simulink model "DA40_Flight_Model"  (R2023a)
settings: Solver=FixedStepAuto  StartTime=DCAM.startTime  StopTime=DCAM.endTime  FixedStep=DCAM.timeStep  RelTol=1e-3
undefined symbols (not defined in the file or in its folder): DCAM, Earth, WGS84
libraries: simulink x27, slpidlib x15, simulink_extras x6, sharedtransform x4, aerolibtransform2 x4, aerolibatmos2 x3, uavalgslib x2, aerolibwind2 x1
(part 2 of 6)

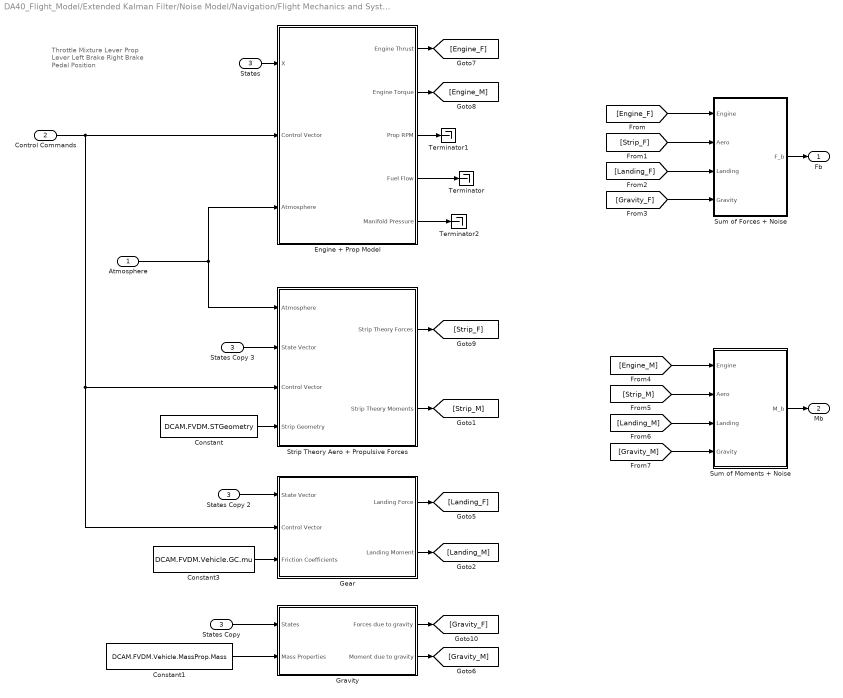
== system DA40_Flight_Model/Extended Kalman Filter/Noise Model/Navigation/Flight Mechanics and Systems Models ==
  note: Throttle
      | Mixture Lever
      | Prop Lever
      | Left Brake
      | Right Brake
      | Pedal Position
  Atmosphere : Inport
  Control Commands : Inport  Port=2
  States : Inport  Port=3
  Constant : Constant  Value=DCAM.FVDM.STGeometry
  Constant1 : Constant  Value=DCAM.FVDM.Vehicle.MassProp.Mass
  Constant3 : Constant  Value=DCAM.FVDM.Vehicle.GC.mu
  Engine + Prop Model : Subsystem
  Gear : Subsystem
  Gravity : Subsystem
  States Copy : InportShadow  Port=3
  States Copy 2 : InportShadow  Port=3
  States Copy 3 : InportShadow  Port=3
  Strip Theory Aero + Propulsive Forces : Subsystem
  Sum of Forces + Noise : Subsystem
  Sum of Moments + Noise : Subsystem
  Terminator : Terminator
  Terminator1 : Terminator
  Terminator2 : Terminator
  Fb : Outport
  Mb : Outport  Port=2
  wires:
  States/1 -> Engine + Prop Model/1(X)
  Constant1/1 -> Gravity/2(Mass Properties)
  Constant/1 -> Strip Theory Aero + Propulsive Forces/4(Strip Geometry)
  Engine + Prop Model/5(Manifold Pressure) -> Terminator2/1
  Engine + Prop Model/3(Prop RPM) -> Terminator1/1
  Constant3/1 -> Gear/3(Friction Coefficients)
  States Copy/1 -> Gravity/1(States)
  States Copy 2/1 -> Gear/1(State Vector)
  States Copy 3/1 -> Strip Theory Aero + Propulsive Forces/2(State Vector)
  Control Commands/1 -> Strip Theory Aero + Propulsive Forces/3(Control Vector), Gear/2(Control Vector), Engine + Prop Model/2(Control Vector)
  Engine + Prop Model/2(Engine Torque) -> [Engine_M]
  Strip Theory Aero + Propulsive Forces/2(Strip Theory Moments) -> [Strip_M]
  Gear/2(Landing Moment) -> [Landing_M]
  Gravity/2(Moment due to gravity) -> [Gravity_M]
  Gravity/1(Forces due to gravity) -> [Gravity_F]
  Gear/1(Landing Force) -> [Landing_F]
  Strip Theory Aero + Propulsive Forces/1(Strip Theory Forces) -> [Strip_F]
  Engine + Prop Model/1(Engine Thrust) -> [Engine_F]
  Sum of Forces + Noise/1(F_b) -> Fb/1
  [Engine_M] -> Sum of Moments + Noise/1(Engine)
  [Strip_M] -> Sum of Moments + Noise/2(Aero)
  [Landing_M] -> Sum of Moments + Noise/3(Landing)
  [Gravity_M] -> Sum of Moments + Noise/4(Gravity)
  Atmosphere/1 -> Strip Theory Aero + Propulsive Forces/1(Atmosphere), Engine + Prop Model/3(Atmosphere)
  Engine + Prop Model/4(Fuel Flow) -> Terminator/1
  [Gravity_F] -> Sum of Forces + Noise/4(Gravity)
  [Landing_F] -> Sum of Forces + Noise/3(Landing)
  [Strip_F] -> Sum of Forces + Noise/2(Aero)
  [Engine_F] -> Sum of Forces + Noise/1(Engine)
  Sum of Moments + Noise/1(M_b) -> Mb/1

== system DA40_Flight_Model/Correlator Simulation/Subsystem1/Generating GPS and Satellite Measurements/Truth Model/Control ==
  Commands : Inport
  States : Inport  Port=2
  Atmos : Inport  Port=3
  Bus Creator : BusCreator  Inputs=12
  Bus Selector : BusSelector  OutputSignals=Commanded Pitch,Commanded Bank,Commanded Velocity,Commanded Propeller Efficiency,Commanded Fuel Mixture,Commanded Flap Angle,Commanded Left Brake,Commanded Right Brake,Commanded Aileron Trim,Commanded Elevator Trim,Commanded Rudder Trim
  Send To Workspace : Subsystem
      settings: PortSchema="{\"entries\":[{\"content\":{\"sides\":[{\"content\":{\"connectorIds\":[\"In1\"]},\"type\":\"ConnectorPlacement.EquallySpacedRectSide\",\"uuid\":\"f8d70518-feba-4467-9144-e72499141e10\"},{\"content\":{\"connectorIds\":[\"Out1\"],\"side\":\"RIGHT\"},\"type\":\"ConnectorPlacement.EquallySpacedRectSide\",\"uuid\":\"0d837ca8-6650-40ee-933a-3521e14176de\"},{\"content\":{\"side\":\"TOP\"},\"type\":\"ConnectorPlacement.EquallySpacedRectSide\",\"uuid\":\"54f7b60b-7724-46f0-8f38-219401d515c7\"},{\"content\":{\"connectorIds\":[\"Out2\"],\"side\":\"BOTTOM\"},\"type\":\"ConnectorPlacement.EquallySpacedRectSide\",\"uuid\":\"f1e71b5c-4796-4085-9245-75f71ccb39d6\"}]},\"type\":\"ConnectorPlacement.EquallySpacedConnector\",\"uuid\":\"946e06f8-2adb-45c5-9153-0b4b2f8d0bb6\"}],\"packageUris\":[\"http://schema.mathworks.com/mf0/Connector/R2020b\"],\"version\":\"1.0\"}"
  Subsystem : Subsystem
      settings: PortSchema="{\"entries\":[{\"content\":{\"sides\":[{\"content\":{\"connectorIds\":[\"In1\"]},\"type\":\"ConnectorPlacement.EquallySpacedRectSide\",\"uuid\":\"5ea7349d-baf6-49c5-809d-4b912ce56d76\"},{\"content\":{\"connectorIds\":[\"Out1\",\"Out2\"],\"side\":\"RIGHT\"},\"type\":\"ConnectorPlacement.EquallySpacedRectSide\",\"uuid\":\"ab3ceec7-e245-42b0-9eb8-e3a68951e219\"},{\"content\":{\"connectorIds\":[\"In2\"],\"side\":\"TOP\"},\"type\":\"ConnectorPlacement.EquallySpacedRectSide\",\"uuid\":\"18178c43-0035-4aec-a3ba-011af3830f5c\"},{\"content\":{\"connectorIds\":[\"Out3\"],\"side\":\"BOTTOM\"},\"type\":\"ConnectorPlacement.EquallySpacedRectSide\",\"uuid\":\"88476787-2df8-4308-98f2-16231590cef9\"}]},\"type\":\"ConnectorPlacement.EquallySpacedConnector\",\"uuid\":\"0f7476f8-a4e6-4d2f-9698-249fd1b1cc90\"}],\"packageUris\":[\"http://schema.mathworks.com/mf0/Connector/R2020b\"],\"version\":\"1.0\"}"
  Subsystem1 : Subsystem
      settings: PortSchema="{\"entries\":[{\"content\":{\"sides\":[{\"content\":{\"connectorIds\":[\"In1\"]},\"type\":\"ConnectorPlacement.EquallySpacedRectSide\",\"uuid\":\"df1e81ab-d97f-43f0-8cd1-ba06c25288e8\"},{\"content\":{\"connectorIds\":[\"Out1\"],\"side\":\"RIGHT\"},\"type\":\"ConnectorPlacement.EquallySpacedRectSide\",\"uuid\":\"fe7f65be-8a13-42ab-8ffa-afe418a633fa\"},{\"content\":{\"connectorIds\":[\"In2\"],\"side\":\"TOP\"},\"type\":\"ConnectorPlacement.EquallySpacedRectSide\",\"uuid\":\"4762097a-1dfd-4646-aeb3-678774417eb9\"},{\"content\":{\"connectorIds\":[\"Out2\"],\"side\":\"BOTTOM\"},\"type\":\"ConnectorPlacement.EquallySpacedRectSide\",\"uuid\":\"338e28fc-4594-4f48-8379-f1c16de78061\"}]},\"type\":\"ConnectorPlacement.EquallySpacedConnector\",\"uuid\":\"e1e6a329-5243-44ef-b6a4-a2802fff17f2\"}],\"packageUris\":[\"http://schema.mathworks.com/mf0/Connector/R2020b\"],\"version\":\"1.0\"}"
  Subsystem10 : Subsystem
      settings: PortSchema="{\"entries\":[{\"content\":{\"sides\":[{\"content\":{\"connectorIds\":[\"In1\"]},\"type\":\"ConnectorPlacement.EquallySpacedRectSide\",\"uuid\":\"df1e81ab-d97f-43f0-8cd1-ba06c25288e8\"},{\"content\":{\"connectorIds\":[\"Out1\"],\"side\":\"RIGHT\"},\"type\":\"ConnectorPlacement.EquallySpacedRectSide\",\"uuid\":\"fe7f65be-8a13-42ab-8ffa-afe418a633fa\"},{\"content\":{\"connectorIds\":[\"In2\"],\"side\":\"TOP\"},\"type\":\"ConnectorPlacement.EquallySpacedRectSide\",\"uuid\":\"4762097a-1dfd-4646-aeb3-678774417eb9\"},{\"content\":{\"connectorIds\":[\"Out2\"],\"side\":\"BOTTOM\"},\"type\":\"ConnectorPlacement.EquallySpacedRectSide\",\"uuid\":\"ca232b1a-28ac-4e7a-b8a6-76103b2c6113\"}]},\"type\":\"ConnectorPlacement.EquallySpacedConnector\",\"uuid\":\"e1e6a329-5243-44ef-b6a4-a2802fff17f2\"}],\"packageUris\":[\"http://schema.mathworks.com/mf0/Connector/R2020b\"],\"version\":\"1.0\"}"
  Subsystem11 : Subsystem
      settings: PortSchema="{\"entries\":[{\"content\":{\"sides\":[{\"content\":{\"connectorIds\":[\"In1\"]},\"type\":\"ConnectorPlacement.EquallySpacedRectSide\",\"uuid\":\"df1e81ab-d97f-43f0-8cd1-ba06c25288e8\"},{\"content\":{\"connectorIds\":[\"Out1\"],\"side\":\"RIGHT\"},\"type\":\"ConnectorPlacement.EquallySpacedRectSide\",\"uuid\":\"fe7f65be-8a13-42ab-8ffa-afe418a633fa\"},{\"content\":{\"connectorIds\":[\"In2\"],\"side\":\"TOP\"},\"type\":\"ConnectorPlacement.EquallySpacedRectSide\",\"uuid\":\"4762097a-1dfd-4646-aeb3-678774417eb9\"}]},\"type\":\"ConnectorPlacement.EquallySpacedConnector\",\"uuid\":\"e1e6a329-5243-44ef-b6a4-a2802fff17f2\"}],\"packageUris\":[\"http://schema.mathworks.com/mf0/Connector/R2020b\"],\"version\":\"1.0\"}"
  Subsystem3 : Subsystem
      settings: PortSchema="{\"entries\":[{\"content\":{\"sides\":[{\"content\":{\"connectorIds\":[\"In1\"]},\"type\":\"ConnectorPlacement.EquallySpacedRectSide\",\"uuid\":\"df1e81ab-d97f-43f0-8cd1-ba06c25288e8\"},{\"content\":{\"connectorIds\":[\"Out1\"],\"side\":\"RIGHT\"},\"type\":\"ConnectorPlacement.EquallySpacedRectSide\",\"uuid\":\"fe7f65be-8a13-42ab-8ffa-afe418a633fa\"},{\"content\":{\"connectorIds\":[\"In2\"],\"side\":\"TOP\"},\"type\":\"ConnectorPlacement.EquallySpacedRectSide\",\"uuid\":\"4762097a-1dfd-4646-aeb3-678774417eb9\"},{\"content\":{\"connectorIds\":[\"Out2\"],\"side\":\"BOTTOM\"},\"type\":\"ConnectorPlacement.EquallySpacedRectSide\",\"uuid\":\"eb7acd08-7b98-4b28-a61a-3ca4385205ec\"}]},\"type\":\"ConnectorPlacement.EquallySpacedConnector\",\"uuid\":\"e1e6a329-5243-44ef-b6a4-a2802fff17f2\"}],\"packageUris\":[\"http://schema.mathworks.com/mf0/Connector/R2020b\"],\"version\":\"1.0\"}"
  Subsystem4 : Subsystem
      settings: PortSchema="{\"entries\":[{\"content\":{\"sides\":[{\"content\":{\"connectorIds\":[\"In1\"]},\"type\":\"ConnectorPlacement.EquallySpacedRectSide\",\"uuid\":\"df1e81ab-d97f-43f0-8cd1-ba06c25288e8\"},{\"content\":{\"connectorIds\":[\"Out1\"],\"side\":\"RIGHT\"},\"type\":\"ConnectorPlacement.EquallySpacedRectSide\",\"uuid\":\"fe7f65be-8a13-42ab-8ffa-afe418a633fa\"},{\"content\":{\"connectorIds\":[\"In2\"],\"side\":\"TOP\"},\"type\":\"ConnectorPlacement.EquallySpacedRectSide\",\"uuid\":\"4762097a-1dfd-4646-aeb3-678774417eb9\"},{\"content\":{\"connectorIds\":[\"Out2\"],\"side\":\"BOTTOM\"},\"type\":\"ConnectorPlacement.EquallySpacedRectSide\",\"uuid\":\"aca1bd27-9370-4c71-9435-0c269f9a438b\"}]},\"type\":\"ConnectorPlacement.EquallySpacedConnector\",\"uuid\":\"e1e6a329-5243-44ef-b6a4-a2802fff17f2\"}],\"packageUris\":[\"http://schema.mathworks.com/mf0/Connector/R2020b\"],\"version\":\"1.0\"}"
  Subsystem5 : Subsystem
      settings: PortSchema="{\"entries\":[{\"content\":{\"sides\":[{\"content\":{\"connectorIds\":[\"In1\"]},\"type\":\"ConnectorPlacement.EquallySpacedRectSide\",\"uuid\":\"df1e81ab-d97f-43f0-8cd1-ba06c25288e8\"},{\"content\":{\"connectorIds\":[\"Out1\"],\"side\":\"RIGHT\"},\"type\":\"ConnectorPlacement.EquallySpacedRectSide\",\"uuid\":\"fe7f65be-8a13-42ab-8ffa-afe418a633fa\"},{\"content\":{\"connectorIds\":[\"In2\"],\"side\":\"TOP\"},\"type\":\"ConnectorPlacement.EquallySpacedRectSide\",\"uuid\":\"4762097a-1dfd-4646-aeb3-678774417eb9\"},{\"content\":{\"connectorIds\":[\"Out2\"],\"side\":\"BOTTOM\"},\"type\":\"ConnectorPlacement.EquallySpacedRectSide\",\"uuid\":\"e3132084-5e8e-4693-9249-2c258902bcf1\"}]},\"type\":\"ConnectorPlacement.EquallySpacedConnector\",\"uuid\":\"e1e6a329-5243-44ef-b6a4-a2802fff17f2\"}],\"packageUris\":[\"http://schema.mathworks.com/mf0/Connector/R2020b\"],\"version\":\"1.0\"}"
  Subsystem6 : Subsystem
      settings: PortSchema="{\"entries\":[{\"content\":{\"sides\":[{\"content\":{\"connectorIds\":[\"In1\"]},\"type\":\"ConnectorPlacement.EquallySpacedRectSide\",\"uuid\":\"df1e81ab-d97f-43f0-8cd1-ba06c25288e8\"},{\"content\":{\"connectorIds\":[\"Out1\"],\"side\":\"RIGHT\"},\"type\":\"ConnectorPlacement.EquallySpacedRectSide\",\"uuid\":\"fe7f65be-8a13-42ab-8ffa-afe418a633fa\"},{\"content\":{\"connectorIds\":[\"In2\"],\"side\":\"TOP\"},\"type\":\"ConnectorPlacement.EquallySpacedRectSide\",\"uuid\":\"4762097a-1dfd-4646-aeb3-678774417eb9\"},{\"content\":{\"connectorIds\":[\"Out2\"],\"side\":\"BOTTOM\"},\"type\":\"ConnectorPlacement.EquallySpacedRectSide\",\"uuid\":\"44b8b4cf-3de4-40e9-9bc3-b7b2ed15b9c4\"}]},\"type\":\"ConnectorPlacement.EquallySpacedConnector\",\"uuid\":\"e1e6a329-5243-44ef-b6a4-a2802fff17f2\"}],\"packageUris\":[\"http://schema.mathworks.com/mf0/Connector/R2020b\"],\"version\":\"1.0\"}"
  Subsystem7 : Subsystem
      settings: PortSchema="{\"entries\":[{\"content\":{\"sides\":[{\"content\":{\"connectorIds\":[\"In1\"]},\"type\":\"ConnectorPlacement.EquallySpacedRectSide\",\"uuid\":\"df1e81ab-d97f-43f0-8cd1-ba06c25288e8\"},{\"content\":{\"connectorIds\":[\"Out1\"],\"side\":\"RIGHT\"},\"type\":\"ConnectorPlacement.EquallySpacedRectSide\",\"uuid\":\"fe7f65be-8a13-42ab-8ffa-afe418a633fa\"},{\"content\":{\"connectorIds\":[\"In2\"],\"side\":\"TOP\"},\"type\":\"ConnectorPlacement.EquallySpacedRectSide\",\"uuid\":\"4762097a-1dfd-4646-aeb3-678774417eb9\"},{\"content\":{\"connectorIds\":[\"Out2\"],\"side\":\"BOTTOM\"},\"type\":\"ConnectorPlacement.EquallySpacedRectSide\",\"uuid\":\"4aea28e3-05ae-492c-9523-17787d8052fd\"}]},\"type\":\"ConnectorPlacement.EquallySpacedConnector\",\"uuid\":\"e1e6a329-5243-44ef-b6a4-a2802fff17f2\"}],\"packageUris\":[\"http://schema.mathworks.com/mf0/Connector/R2020b\"],\"version\":\"1.0\"}"
  Subsystem8 : Subsystem
      settings: PortSchema="{\"entries\":[{\"content\":{\"sides\":[{\"content\":{\"connectorIds\":[\"In1\"]},\"type\":\"ConnectorPlacement.EquallySpacedRectSide\",\"uuid\":\"df1e81ab-d97f-43f0-8cd1-ba06c25288e8\"},{\"content\":{\"connectorIds\":[\"Out1\"],\"side\":\"RIGHT\"},\"type\":\"ConnectorPlacement.EquallySpacedRectSide\",\"uuid\":\"fe7f65be-8a13-42ab-8ffa-afe418a633fa\"},{\"content\":{\"connectorIds\":[\"In2\"],\"side\":\"TOP\"},\"type\":\"ConnectorPlacement.EquallySpacedRectSide\",\"uuid\":\"4762097a-1dfd-4646-aeb3-678774417eb9\"},{\"content\":{\"connectorIds\":[\"Out2\"],\"side\":\"BOTTOM\"},\"type\":\"ConnectorPlacement.EquallySpacedRectSide\",\"uuid\":\"60b425fe-182c-41c2-bc4c-aa97cb3d7ccf\"}]},\"type\":\"ConnectorPlacement.EquallySpacedConnector\",\"uuid\":\"e1e6a329-5243-44ef-b6a4-a2802fff17f2\"}],\"packageUris\":[\"http://schema.mathworks.com/mf0/Connector/R2020b\"],\"version\":\"1.0\"}"
  Subsystem9 : Subsystem
      settings: PortSchema="{\"entries\":[{\"content\":{\"sides\":[{\"content\":{\"connectorIds\":[\"In1\"]},\"type\":\"ConnectorPlacement.EquallySpacedRectSide\",\"uuid\":\"df1e81ab-d97f-43f0-8cd1-ba06c25288e8\"},{\"content\":{\"connectorIds\":[\"Out1\"],\"side\":\"RIGHT\"},\"type\":\"ConnectorPlacement.EquallySpacedRectSide\",\"uuid\":\"fe7f65be-8a13-42ab-8ffa-afe418a633fa\"},{\"content\":{\"connectorIds\":[\"In2\"],\"side\":\"TOP\"},\"type\":\"ConnectorPlacement.EquallySpacedRectSide\",\"uuid\":\"4762097a-1dfd-4646-aeb3-678774417eb9\"},{\"content\":{\"connectorIds\":[\"Out2\"],\"side\":\"BOTTOM\"},\"type\":\"ConnectorPlacement.EquallySpacedRectSide\",\"uuid\":\"88e2b07d-9cf7-412b-8368-04827ebf702b\"}]},\"type\":\"ConnectorPlacement.EquallySpacedConnector\",\"uuid\":\"e1e6a329-5243-44ef-b6a4-a2802fff17f2\"}],\"packageUris\":[\"http://schema.mathworks.com/mf0/Connector/R2020b\"],\"version\":\"1.0\"}"
  To Workspace : ToWorkspace  VariableName=controls  SampleTime=-1
      settings: Save2DSignal=2-D array (concatenate along first dimension)
  Controls : Outport
  Atmosphere : Outport  Port=2
  LLA : Outport  Port=3
  wires:
  Subsystem11/1(Out1) -> Bus Creator/12  "RUDDER TRIM"
  Subsystem9/1(Out1) -> Bus Creator/10  "AILERON TRIM"
  Subsystem1/1(Longitudinal Stick) -> Bus Creator/1  "Longitudinal Stick"
  Subsystem/1(Lateral Stick) -> Bus Creator/2  "Lateral Stick"
  Subsystem6/1(Out1) -> Bus Creator/7  "FLAP ANGLE"
  Subsystem5/1(Out1) -> Bus Creator/6  "Mixture Lever"
  Subsystem3/1(Out1) -> Bus Creator/4  "Throttle"
  Subsystem8/1(Out1) -> Bus Creator/9  "RightBrake"
  Subsystem/2(Pedal Posn) -> Bus Creator/3  "Pedal Posn"
  Subsystem4/1(Out1) -> Bus Creator/5  "Prop Lever"
  Subsystem7/1(Out1) -> Bus Creator/8  "LeftBrake"
  Subsystem10/1(Out1) -> Bus Creator/11  "ELEVATOR TRIM"
  Bus Creator/1 -> To Workspace/1, Controls/1
  Commands/1 -> Bus Selector/1
  Bus Selector/11 -> Subsystem11/1(Reference)  "<Commanded Rudder Trim>"
  Bus Selector/10 -> Subsystem10/1(Reference)  "<Commanded Elevator Trim>"
  Bus Selector/9 -> Subsystem9/1(Reference)  "<Commanded Aileron Trim>"
  Bus Selector/8 -> Subsystem8/1(Reference)  "<Commanded Right Brake>"
  Bus Selector/7 -> Subsystem7/1(Reference)  "<Commanded Left Brake>"
  Bus Selector/6 -> Subsystem6/1(Reference)  "<Commanded Flap Angle>"
  Bus Selector/5 -> Subsystem5/1(Reference)  "<Commanded Fuel Mixture>"
  Bus Selector/4 -> Subsystem4/1(Reference)  "<Commanded Propeller Efficiency>"
  Bus Selector/3 -> Subsystem3/1(Reference)  "<Commanded Velocity>"
  Bus Selector/1 -> Subsystem1/1(Reference)  "<Commanded Pitch>"
  Bus Selector/2 -> Subsystem/1(Reference)  "<Commanded Bank>"
  States/1 -> Send To Workspace/1(States)
  Send To Workspace/2(States Out) -> Subsystem1/2(States)
  Subsystem6/2(" ") -> Subsystem7/2(States)
  Subsystem9/2(" ") -> Subsystem10/2(States)
  Subsystem3/2(" ") -> Subsystem4/2(States)
  Subsystem/3(" ") -> Subsystem3/2(States)
  Subsystem1/2(" ") -> Subsystem/2(States)
  Subsystem7/2(" ") -> Subsystem8/2(States)
  Subsystem8/2(" ") -> Subsystem9/2(States)
  Subsystem5/2(" ") -> Subsystem6/2(States)
  Subsystem4/2(" ") -> Subsystem5/2(States)
  Subsystem10/2(" ") -> Subsystem11/2(States)
  Atmos/1 -> Atmosphere/1
  Send To Workspace/1(LLA) -> LLA/1

== system DA40_Flight_Model/Correlator Simulation/Subsystem1/Generating GPS and Satellite Measurements/Truth Model/Environment ==
  States : Inport
  LLA : Inport  Port=2
  Bus Creator : BusCreator  Inputs=5
  Clock : Clock
  Constant1 : Constant  Value=DCAM.FVDM.dayOfYear
  Gain1 : Gain  Gain=-1
  Horizontal Wind Model 14 : WindHWM14
  ISA Atmosphere Model : aerolibatmos2/ISA Atmosphere Model  custom=off  g=9.80665  gamma=1.4  R=287.0531  L=0.0065  h_trop=11000  h_strat=20000  rho0=1.225  P0=101325  T0=288.15  h0=0
  MATLAB Function : MATLAB Function  TreatAsAtomicUnit=on
  Selector1 : Selector  InputPortWidth=12  IndexOptions=Index vector (dialog)  Indices=[9]  OutputSizes=1
  States Out : Outport
  Atmos : Outport  Port=2
  wires:
  States/1 -> MATLAB Function/2(states), States Out/1, Selector1/1
  Selector1/1 -> Gain1/1
  ISA Atmosphere Model/2 -> Bus Creator/2  "Speed of Sound"
  ISA Atmosphere Model/3 -> Bus Creator/3  "Pressure"
  Bus Creator/1 -> Atmos/1
  ISA Atmosphere Model/1 -> Bus Creator/1  "Temperature"
  Gain1/1 -> ISA Atmosphere Model/1
  ISA Atmosphere Model/4 -> Bus Creator/4  "Density"
  LLA/1 -> Horizontal Wind Model 14/1
  Clock/1 -> Horizontal Wind Model 14/3
  Constant1/1 -> Horizontal Wind Model 14/2
  Horizontal Wind Model 14/1 -> MATLAB Function/1(windVectorNav)  "Wind Vector"
  MATLAB Function/1(windVectorBody) -> Bus Creator/5

== system DA40_Flight_Model/Correlator Simulation/Subsystem1/Generating GPS and Satellite Measurements/Truth Model/Guidance ==
  States : Inport
  Atmosphere : Inport  Port=2
  Bus Creator : BusCreator  Inputs=11
  Bus Selector : BusSelector  OutputSignals=x,y,z,psi
  Constant : Constant  Value=DCAM.FVDM.waypoints
  Constant1 : Constant  Value=DCAM.FVDM.lookaheadDist
  MATLAB Function : MATLAB Function  TreatAsAtomicUnit=on
  Mux : Mux
  Radians to Degrees : simulink_extras/Transformations/Radians to Degrees
  Subsystem : Subsystem
  Terminator : Terminator
  Terminator1 : Terminator
  Waypoint Follower : uavalgslib/Waypoint Follower  UAVType=fixed-wing  StartFrom=first  TransitionRadiusSource=internal  TransitionRadius=10  MinLookaheadDistance=0.1  YawInput=off  ShowCrossTrackErrorOutput=off  ShowStatusOutput=off  SimulateUsing=Code generation
  Commands : Outport
  States Out : Outport  Port=2
  Atmos : Outport  Port=3
  wires:
  Bus Creator/1 -> Commands/1
  Subsystem/1(Bank) -> Bus Creator/1  "Commanded Bank"
  Subsystem/2(Pitch) -> Bus Creator/2  "Commanded Pitch"
  Subsystem/3(Velocity) -> Bus Creator/3  "Commanded Velocity"
  Subsystem/4(Propeller Efficiency) -> Bus Creator/4  "Commanded Propeller Efficiency"
  Subsystem/5(Fuel Efficiency) -> Bus Creator/5  "Commanded Fuel Mixture"
  Subsystem/6(Flap Angle) -> Bus Creator/6  "Commanded Flap Angle"
  Subsystem/7(Left Brake) -> Bus Creator/7  "Commanded Left Brake"
  Subsystem/8(Right Brake) -> Bus Creator/8  "Commanded Right Brake"
  Subsystem/9(Aileron trim) -> Bus Creator/9  "Commanded Aileron Trim"
  Subsystem/10(Elevator Trim) -> Bus Creator/10  "Commanded Elevator Trim"
  Subsystem/11(Rudder Trim) -> Bus Creator/11  "Commanded Rudder Trim"
  States/1 -> Bus Selector/1, States Out/1
  Waypoint Follower/3 -> Terminator/1
  Waypoint Follower/4 -> Terminator1/1
  Constant/1 -> Waypoint Follower/2
  Constant1/1 -> Waypoint Follower/3
  Mux/1 -> Waypoint Follower/1
  Bus Selector/1 -> Mux/1  "<x>"
  Bus Selector/2 -> Mux/2  "<y>"
  Bus Selector/3 -> Mux/3  "<z>"
  Waypoint Follower/2 -> MATLAB Function/1("heading ")
  Atmosphere/1 -> Atmos/1
  Waypoint Follower/1 -> Subsystem/1(Target)
  MATLAB Function/1(heading) -> Subsystem/2(Desired Heading)
  Radians to Degrees/1 -> Mux/4, Subsystem/3(Heading)
  Bus Selector/4 -> Radians to Degrees/1  "<psi>"

== system DA40_Flight_Model/Correlator Simulation/Subsystem1/Generating GPS and Satellite Measurements/Truth Model/Navigation1 ==
  Atmosphere : Inport
  Controls : Inport  Port=2
  Constant1 : Constant  Value=DCAM.FVDM.Vehicle.MassProp.Mass
  DA-40 Equations of Motion : Subsystem
  Flight Mechanics and Systems Models : Subsystem
  States : Outport
  wires:
  Flight Mechanics and Systems Models/1(Fb) -> DA-40 Equations of Motion/1(Fb [lb])
  Flight Mechanics and Systems Models/2(Mb) -> DA-40 Equations of Motion/2(Mb [lb-ft])
  Controls/1 -> Flight Mechanics and Systems Models/2(Control Commands)
  Atmosphere/1 -> Flight Mechanics and Systems Models/1(Atmosphere)
  Constant1/1 -> DA-40 Equations of Motion/3(Mass Properties)
  DA-40 Equations of Motion/1(States) -> States/1, Flight Mechanics and Systems Models/3(States)

== system DA40_Flight_Model/Correlator Simulation/Subsystem1/Generating GPS and Satellite Measurements1/Truth Model/Control ==
  Commands : Inport
  States : Inport  Port=2
  Atmos : Inport  Port=3
  Bus Creator : BusCreator  Inputs=12
  Bus Selector : BusSelector  OutputSignals=Commanded Pitch,Commanded Bank,Commanded Velocity,Commanded Propeller Efficiency,Commanded Fuel Mixture,Commanded Flap Angle,Commanded Left Brake,Commanded Right Brake,Commanded Aileron Trim,Commanded Elevator Trim,Commanded Rudder Trim
  Send To Workspace : Subsystem
      settings: PortSchema="{\"entries\":[{\"content\":{\"sides\":[{\"content\":{\"connectorIds\":[\"In1\"]},\"type\":\"ConnectorPlacement.EquallySpacedRectSide\",\"uuid\":\"f8d70518-feba-4467-9144-e72499141e10\"},{\"content\":{\"connectorIds\":[\"Out1\"],\"side\":\"RIGHT\"},\"type\":\"ConnectorPlacement.EquallySpacedRectSide\",\"uuid\":\"0d837ca8-6650-40ee-933a-3521e14176de\"},{\"content\":{\"side\":\"TOP\"},\"type\":\"ConnectorPlacement.EquallySpacedRectSide\",\"uuid\":\"54f7b60b-7724-46f0-8f38-219401d515c7\"},{\"content\":{\"connectorIds\":[\"Out2\"],\"side\":\"BOTTOM\"},\"type\":\"ConnectorPlacement.EquallySpacedRectSide\",\"uuid\":\"f1e71b5c-4796-4085-9245-75f71ccb39d6\"}]},\"type\":\"ConnectorPlacement.EquallySpacedConnector\",\"uuid\":\"946e06f8-2adb-45c5-9153-0b4b2f8d0bb6\"}],\"packageUris\":[\"http://schema.mathworks.com/mf0/Connector/R2020b\"],\"version\":\"1.0\"}"
  Subsystem : Subsystem
      settings: PortSchema="{\"entries\":[{\"content\":{\"sides\":[{\"content\":{\"connectorIds\":[\"In1\"]},\"type\":\"ConnectorPlacement.EquallySpacedRectSide\",\"uuid\":\"5ea7349d-baf6-49c5-809d-4b912ce56d76\"},{\"content\":{\"connectorIds\":[\"Out1\",\"Out2\"],\"side\":\"RIGHT\"},\"type\":\"ConnectorPlacement.EquallySpacedRectSide\",\"uuid\":\"ab3ceec7-e245-42b0-9eb8-e3a68951e219\"},{\"content\":{\"connectorIds\":[\"In2\"],\"side\":\"TOP\"},\"type\":\"ConnectorPlacement.EquallySpacedRectSide\",\"uuid\":\"18178c43-0035-4aec-a3ba-011af3830f5c\"},{\"content\":{\"connectorIds\":[\"Out3\"],\"side\":\"BOTTOM\"},\"type\":\"ConnectorPlacement.EquallySpacedRectSide\",\"uuid\":\"88476787-2df8-4308-98f2-16231590cef9\"}]},\"type\":\"ConnectorPlacement.EquallySpacedConnector\",\"uuid\":\"0f7476f8-a4e6-4d2f-9698-249fd1b1cc90\"}],\"packageUris\":[\"http://schema.mathworks.com/mf0/Connector/R2020b\"],\"version\":\"1.0\"}"
  Subsystem1 : Subsystem
      settings: PortSchema="{\"entries\":[{\"content\":{\"sides\":[{\"content\":{\"connectorIds\":[\"In1\"]},\"type\":\"ConnectorPlacement.EquallySpacedRectSide\",\"uuid\":\"df1e81ab-d97f-43f0-8cd1-ba06c25288e8\"},{\"content\":{\"connectorIds\":[\"Out1\"],\"side\":\"RIGHT\"},\"type\":\"ConnectorPlacement.EquallySpacedRectSide\",\"uuid\":\"fe7f65be-8a13-42ab-8ffa-afe418a633fa\"},{\"content\":{\"connectorIds\":[\"In2\"],\"side\":\"TOP\"},\"type\":\"ConnectorPlacement.EquallySpacedRectSide\",\"uuid\":\"4762097a-1dfd-4646-aeb3-678774417eb9\"},{\"content\":{\"connectorIds\":[\"Out2\"],\"side\":\"BOTTOM\"},\"type\":\"ConnectorPlacement.EquallySpacedRectSide\",\"uuid\":\"338e28fc-4594-4f48-8379-f1c16de78061\"}]},\"type\":\"ConnectorPlacement.EquallySpacedConnector\",\"uuid\":\"e1e6a329-5243-44ef-b6a4-a2802fff17f2\"}],\"packageUris\":[\"http://schema.mathworks.com/mf0/Connector/R2020b\"],\"version\":\"1.0\"}"
  Subsystem10 : Subsystem
      settings: PortSchema="{\"entries\":[{\"content\":{\"sides\":[{\"content\":{\"connectorIds\":[\"In1\"]},\"type\":\"ConnectorPlacement.EquallySpacedRectSide\",\"uuid\":\"df1e81ab-d97f-43f0-8cd1-ba06c25288e8\"},{\"content\":{\"connectorIds\":[\"Out1\"],\"side\":\"RIGHT\"},\"type\":\"ConnectorPlacement.EquallySpacedRectSide\",\"uuid\":\"fe7f65be-8a13-42ab-8ffa-afe418a633fa\"},{\"content\":{\"connectorIds\":[\"In2\"],\"side\":\"TOP\"},\"type\":\"ConnectorPlacement.EquallySpacedRectSide\",\"uuid\":\"4762097a-1dfd-4646-aeb3-678774417eb9\"},{\"content\":{\"connectorIds\":[\"Out2\"],\"side\":\"BOTTOM\"},\"type\":\"ConnectorPlacement.EquallySpacedRectSide\",\"uuid\":\"ca232b1a-28ac-4e7a-b8a6-76103b2c6113\"}]},\"type\":\"ConnectorPlacement.EquallySpacedConnector\",\"uuid\":\"e1e6a329-5243-44ef-b6a4-a2802fff17f2\"}],\"packageUris\":[\"http://schema.mathworks.com/mf0/Connector/R2020b\"],\"version\":\"1.0\"}"
  Subsystem11 : Subsystem
      settings: PortSchema="{\"entries\":[{\"content\":{\"sides\":[{\"content\":{\"connectorIds\":[\"In1\"]},\"type\":\"ConnectorPlacement.EquallySpacedRectSide\",\"uuid\":\"df1e81ab-d97f-43f0-8cd1-ba06c25288e8\"},{\"content\":{\"connectorIds\":[\"Out1\"],\"side\":\"RIGHT\"},\"type\":\"ConnectorPlacement.EquallySpacedRectSide\",\"uuid\":\"fe7f65be-8a13-42ab-8ffa-afe418a633fa\"},{\"content\":{\"connectorIds\":[\"In2\"],\"side\":\"TOP\"},\"type\":\"ConnectorPlacement.EquallySpacedRectSide\",\"uuid\":\"4762097a-1dfd-4646-aeb3-678774417eb9\"}]},\"type\":\"ConnectorPlacement.EquallySpacedConnector\",\"uuid\":\"e1e6a329-5243-44ef-b6a4-a2802fff17f2\"}],\"packageUris\":[\"http://schema.mathworks.com/mf0/Connector/R2020b\"],\"version\":\"1.0\"}"
  Subsystem3 : Subsystem
      settings: PortSchema="{\"entries\":[{\"content\":{\"sides\":[{\"content\":{\"connectorIds\":[\"In1\"]},\"type\":\"ConnectorPlacement.EquallySpacedRectSide\",\"uuid\":\"df1e81ab-d97f-43f0-8cd1-ba06c25288e8\"},{\"content\":{\"connectorIds\":[\"Out1\"],\"side\":\"RIGHT\"},\"type\":\"ConnectorPlacement.EquallySpacedRectSide\",\"uuid\":\"fe7f65be-8a13-42ab-8ffa-afe418a633fa\"},{\"content\":{\"connectorIds\":[\"In2\"],\"side\":\"TOP\"},\"type\":\"ConnectorPlacement.EquallySpacedRectSide\",\"uuid\":\"4762097a-1dfd-4646-aeb3-678774417eb9\"},{\"content\":{\"connectorIds\":[\"Out2\"],\"side\":\"BOTTOM\"},\"type\":\"ConnectorPlacement.EquallySpacedRectSide\",\"uuid\":\"eb7acd08-7b98-4b28-a61a-3ca4385205ec\"}]},\"type\":\"ConnectorPlacement.EquallySpacedConnector\",\"uuid\":\"e1e6a329-5243-44ef-b6a4-a2802fff17f2\"}],\"packageUris\":[\"http://schema.mathworks.com/mf0/Connector/R2020b\"],\"version\":\"1.0\"}"
  Subsystem4 : Subsystem
      settings: PortSchema="{\"entries\":[{\"content\":{\"sides\":[{\"content\":{\"connectorIds\":[\"In1\"]},\"type\":\"ConnectorPlacement.EquallySpacedRectSide\",\"uuid\":\"df1e81ab-d97f-43f0-8cd1-ba06c25288e8\"},{\"content\":{\"connectorIds\":[\"Out1\"],\"side\":\"RIGHT\"},\"type\":\"ConnectorPlacement.EquallySpacedRectSide\",\"uuid\":\"fe7f65be-8a13-42ab-8ffa-afe418a633fa\"},{\"content\":{\"connectorIds\":[\"In2\"],\"side\":\"TOP\"},\"type\":\"ConnectorPlacement.EquallySpacedRectSide\",\"uuid\":\"4762097a-1dfd-4646-aeb3-678774417eb9\"},{\"content\":{\"connectorIds\":[\"Out2\"],\"side\":\"BOTTOM\"},\"type\":\"ConnectorPlacement.EquallySpacedRectSide\",\"uuid\":\"aca1bd27-9370-4c71-9435-0c269f9a438b\"}]},\"type\":\"ConnectorPlacement.EquallySpacedConnector\",\"uuid\":\"e1e6a329-5243-44ef-b6a4-a2802fff17f2\"}],\"packageUris\":[\"http://schema.mathworks.com/mf0/Connector/R2020b\"],\"version\":\"1.0\"}"
  Subsystem5 : Subsystem
      settings: PortSchema="{\"entries\":[{\"content\":{\"sides\":[{\"content\":{\"connectorIds\":[\"In1\"]},\"type\":\"ConnectorPlacement.EquallySpacedRectSide\",\"uuid\":\"df1e81ab-d97f-43f0-8cd1-ba06c25288e8\"},{\"content\":{\"connectorIds\":[\"Out1\"],\"side\":\"RIGHT\"},\"type\":\"ConnectorPlacement.EquallySpacedRectSide\",\"uuid\":\"fe7f65be-8a13-42ab-8ffa-afe418a633fa\"},{\"content\":{\"connectorIds\":[\"In2\"],\"side\":\"TOP\"},\"type\":\"ConnectorPlacement.EquallySpacedRectSide\",\"uuid\":\"4762097a-1dfd-4646-aeb3-678774417eb9\"},{\"content\":{\"connectorIds\":[\"Out2\"],\"side\":\"BOTTOM\"},\"type\":\"ConnectorPlacement.EquallySpacedRectSide\",\"uuid\":\"e3132084-5e8e-4693-9249-2c258902bcf1\"}]},\"type\":\"ConnectorPlacement.EquallySpacedConnector\",\"uuid\":\"e1e6a329-5243-44ef-b6a4-a2802fff17f2\"}],\"packageUris\":[\"http://schema.mathworks.com/mf0/Connector/R2020b\"],\"version\":\"1.0\"}"
  Subsystem6 : Subsystem
      settings: PortSchema="{\"entries\":[{\"content\":{\"sides\":[{\"content\":{\"connectorIds\":[\"In1\"]},\"type\":\"ConnectorPlacement.EquallySpacedRectSide\",\"uuid\":\"df1e81ab-d97f-43f0-8cd1-ba06c25288e8\"},{\"content\":{\"connectorIds\":[\"Out1\"],\"side\":\"RIGHT\"},\"type\":\"ConnectorPlacement.EquallySpacedRectSide\",\"uuid\":\"fe7f65be-8a13-42ab-8ffa-afe418a633fa\"},{\"content\":{\"connectorIds\":[\"In2\"],\"side\":\"TOP\"},\"type\":\"ConnectorPlacement.EquallySpacedRectSide\",\"uuid\":\"4762097a-1dfd-4646-aeb3-678774417eb9\"},{\"content\":{\"connectorIds\":[\"Out2\"],\"side\":\"BOTTOM\"},\"type\":\"ConnectorPlacement.EquallySpacedRectSide\",\"uuid\":\"44b8b4cf-3de4-40e9-9bc3-b7b2ed15b9c4\"}]},\"type\":\"ConnectorPlacement.EquallySpacedConnector\",\"uuid\":\"e1e6a329-5243-44ef-b6a4-a2802fff17f2\"}],\"packageUris\":[\"http://schema.mathworks.com/mf0/Connector/R2020b\"],\"version\":\"1.0\"}"
  Subsystem7 : Subsystem
      settings: PortSchema="{\"entries\":[{\"content\":{\"sides\":[{\"content\":{\"connectorIds\":[\"In1\"]},\"type\":\"ConnectorPlacement.EquallySpacedRectSide\",\"uuid\":\"df1e81ab-d97f-43f0-8cd1-ba06c25288e8\"},{\"content\":{\"connectorIds\":[\"Out1\"],\"side\":\"RIGHT\"},\"type\":\"ConnectorPlacement.EquallySpacedRectSide\",\"uuid\":\"fe7f65be-8a13-42ab-8ffa-afe418a633fa\"},{\"content\":{\"connectorIds\":[\"In2\"],\"side\":\"TOP\"},\"type\":\"ConnectorPlacement.EquallySpacedRectSide\",\"uuid\":\"4762097a-1dfd-4646-aeb3-678774417eb9\"},{\"content\":{\"connectorIds\":[\"Out2\"],\"side\":\"BOTTOM\"},\"type\":\"ConnectorPlacement.EquallySpacedRectSide\",\"uuid\":\"4aea28e3-05ae-492c-9523-17787d8052fd\"}]},\"type\":\"ConnectorPlacement.EquallySpacedConnector\",\"uuid\":\"e1e6a329-5243-44ef-b6a4-a2802fff17f2\"}],\"packageUris\":[\"http://schema.mathworks.com/mf0/Connector/R2020b\"],\"version\":\"1.0\"}"
  Subsystem8 : Subsystem
      settings: PortSchema="{\"entries\":[{\"content\":{\"sides\":[{\"content\":{\"connectorIds\":[\"In1\"]},\"type\":\"ConnectorPlacement.EquallySpacedRectSide\",\"uuid\":\"df1e81ab-d97f-43f0-8cd1-ba06c25288e8\"},{\"content\":{\"connectorIds\":[\"Out1\"],\"side\":\"RIGHT\"},\"type\":\"ConnectorPlacement.EquallySpacedRectSide\",\"uuid\":\"fe7f65be-8a13-42ab-8ffa-afe418a633fa\"},{\"content\":{\"connectorIds\":[\"In2\"],\"side\":\"TOP\"},\"type\":\"ConnectorPlacement.EquallySpacedRectSide\",\"uuid\":\"4762097a-1dfd-4646-aeb3-678774417eb9\"},{\"content\":{\"connectorIds\":[\"Out2\"],\"side\":\"BOTTOM\"},\"type\":\"ConnectorPlacement.EquallySpacedRectSide\",\"uuid\":\"60b425fe-182c-41c2-bc4c-aa97cb3d7ccf\"}]},\"type\":\"ConnectorPlacement.EquallySpacedConnector\",\"uuid\":\"e1e6a329-5243-44ef-b6a4-a2802fff17f2\"}],\"packageUris\":[\"http://schema.mathworks.com/mf0/Connector/R2020b\"],\"version\":\"1.0\"}"
  Subsystem9 : Subsystem
      settings: PortSchema="{\"entries\":[{\"content\":{\"sides\":[{\"content\":{\"connectorIds\":[\"In1\"]},\"type\":\"ConnectorPlacement.EquallySpacedRectSide\",\"uuid\":\"df1e81ab-d97f-43f0-8cd1-ba06c25288e8\"},{\"content\":{\"connectorIds\":[\"Out1\"],\"side\":\"RIGHT\"},\"type\":\"ConnectorPlacement.EquallySpacedRectSide\",\"uuid\":\"fe7f65be-8a13-42ab-8ffa-afe418a633fa\"},{\"content\":{\"connectorIds\":[\"In2\"],\"side\":\"TOP\"},\"type\":\"ConnectorPlacement.EquallySpacedRectSide\",\"uuid\":\"4762097a-1dfd-4646-aeb3-678774417eb9\"},{\"content\":{\"connectorIds\":[\"Out2\"],\"side\":\"BOTTOM\"},\"type\":\"ConnectorPlacement.EquallySpacedRectSide\",\"uuid\":\"88e2b07d-9cf7-412b-8368-04827ebf702b\"}]},\"type\":\"ConnectorPlacement.EquallySpacedConnector\",\"uuid\":\"e1e6a329-5243-44ef-b6a4-a2802fff17f2\"}],\"packageUris\":[\"http://schema.mathworks.com/mf0/Connector/R2020b\"],\"version\":\"1.0\"}"
  To Workspace : ToWorkspace  VariableName=controls  SampleTime=-1
      settings: Save2DSignal=2-D array (concatenate along first dimension)
  Controls : Outport
  Atmosphere : Outport  Port=2
  LLA : Outport  Port=3
  wires:
  Subsystem11/1(Out1) -> Bus Creator/12  "RUDDER TRIM"
  Subsystem9/1(Out1) -> Bus Creator/10  "AILERON TRIM"
  Subsystem1/1(Longitudinal Stick) -> Bus Creator/1  "Longitudinal Stick"
  Subsystem/1(Lateral Stick) -> Bus Creator/2  "Lateral Stick"
  Subsystem6/1(Out1) -> Bus Creator/7  "FLAP ANGLE"
  Subsystem5/1(Out1) -> Bus Creator/6  "Mixture Lever"
  Subsystem3/1(Out1) -> Bus Creator/4  "Throttle"
  Subsystem8/1(Out1) -> Bus Creator/9  "RightBrake"
  Subsystem/2(Pedal Posn) -> Bus Creator/3  "Pedal Posn"
  Subsystem4/1(Out1) -> Bus Creator/5  "Prop Lever"
  Subsystem7/1(Out1) -> Bus Creator/8  "LeftBrake"
  Subsystem10/1(Out1) -> Bus Creator/11  "ELEVATOR TRIM"
  Bus Creator/1 -> To Workspace/1, Controls/1
  Commands/1 -> Bus Selector/1
  Bus Selector/11 -> Subsystem11/1(Reference)  "<Commanded Rudder Trim>"
  Bus Selector/10 -> Subsystem10/1(Reference)  "<Commanded Elevator Trim>"
  Bus Selector/9 -> Subsystem9/1(Reference)  "<Commanded Aileron Trim>"
  Bus Selector/8 -> Subsystem8/1(Reference)  "<Commanded Right Brake>"
  Bus Selector/7 -> Subsystem7/1(Reference)  "<Commanded Left Brake>"
  Bus Selector/6 -> Subsystem6/1(Reference)  "<Commanded Flap Angle>"
  Bus Selector/5 -> Subsystem5/1(Reference)  "<Commanded Fuel Mixture>"
  Bus Selector/4 -> Subsystem4/1(Reference)  "<Commanded Propeller Efficiency>"
  Bus Selector/3 -> Subsystem3/1(Reference)  "<Commanded Velocity>"
  Bus Selector/1 -> Subsystem1/1(Reference)  "<Commanded Pitch>"
  Bus Selector/2 -> Subsystem/1(Reference)  "<Commanded Bank>"
  States/1 -> Send To Workspace/1(States)
  Send To Workspace/2(States Out) -> Subsystem1/2(States)
  Subsystem6/2(" ") -> Subsystem7/2(States)
  Subsystem9/2(" ") -> Subsystem10/2(States)
  Subsystem3/2(" ") -> Subsystem4/2(States)
  Subsystem/3(" ") -> Subsystem3/2(States)
  Subsystem1/2(" ") -> Subsystem/2(States)
  Subsystem7/2(" ") -> Subsystem8/2(States)
  Subsystem8/2(" ") -> Subsystem9/2(States)
  Subsystem5/2(" ") -> Subsystem6/2(States)
  Subsystem4/2(" ") -> Subsystem5/2(States)
  Subsystem10/2(" ") -> Subsystem11/2(States)
  Atmos/1 -> Atmosphere/1
  Send To Workspace/1(LLA) -> LLA/1

== system DA40_Flight_Model/Correlator Simulation/Subsystem1/Generating GPS and Satellite Measurements1/Truth Model/Environment ==
  States : Inport
  LLA : Inport  Port=2
  Bus Creator : BusCreator  Inputs=5
  Clock : Clock
  Constant1 : Constant  Value=DCAM.FVDM.dayOfYear
  Gain1 : Gain  Gain=-1
  Horizontal Wind Model 14 : WindHWM14
  ISA Atmosphere Model : aerolibatmos2/ISA Atmosphere Model  custom=off  g=9.80665  gamma=1.4  R=287.0531  L=0.0065  h_trop=11000  h_strat=20000  rho0=1.225  P0=101325  T0=288.15  h0=0
  MATLAB Function : MATLAB Function  TreatAsAtomicUnit=on
  Selector1 : Selector  InputPortWidth=12  IndexOptions=Index vector (dialog)  Indices=[9]  OutputSizes=1
  States Out : Outport
  Atmos : Outport  Port=2
  wires:
  States/1 -> MATLAB Function/2(states), States Out/1, Selector1/1
  Selector1/1 -> Gain1/1
  ISA Atmosphere Model/2 -> Bus Creator/2  "Speed of Sound"
  ISA Atmosphere Model/3 -> Bus Creator/3  "Pressure"
  Bus Creator/1 -> Atmos/1
  ISA Atmosphere Model/1 -> Bus Creator/1  "Temperature"
  Gain1/1 -> ISA Atmosphere Model/1
  ISA Atmosphere Model/4 -> Bus Creator/4  "Density"
  LLA/1 -> Horizontal Wind Model 14/1
  Clock/1 -> Horizontal Wind Model 14/3
  Constant1/1 -> Horizontal Wind Model 14/2
  Horizontal Wind Model 14/1 -> MATLAB Function/1(windVectorNav)  "Wind Vector"
  MATLAB Function/1(windVectorBody) -> Bus Creator/5

== system DA40_Flight_Model/Correlator Simulation/Subsystem1/Generating GPS and Satellite Measurements1/Truth Model/Guidance ==
  States : Inport
  Atmosphere : Inport  Port=2
  Bus Creator : BusCreator  Inputs=11
  Bus Selector : BusSelector  OutputSignals=x,y,z,psi
  Constant : Constant  Value=DCAM.FVDM.waypoints
  Constant1 : Constant  Value=DCAM.FVDM.lookaheadDist
  MATLAB Function : MATLAB Function  TreatAsAtomicUnit=on
  Mux : Mux
  Radians to Degrees : simulink_extras/Transformations/Radians to Degrees
  Subsystem : Subsystem
  Terminator : Terminator
  Terminator1 : Terminator
  Waypoint Follower : uavalgslib/Waypoint Follower  UAVType=fixed-wing  StartFrom=first  TransitionRadiusSource=internal  TransitionRadius=10  MinLookaheadDistance=0.1  YawInput=off  ShowCrossTrackErrorOutput=off  ShowStatusOutput=off  SimulateUsing=Code generation
  Commands : Outport
  States Out : Outport  Port=2
  Atmos : Outport  Port=3
  wires:
  Bus Creator/1 -> Commands/1
  Subsystem/1(Bank) -> Bus Creator/1  "Commanded Bank"
  Subsystem/2(Pitch) -> Bus Creator/2  "Commanded Pitch"
  Subsystem/3(Velocity) -> Bus Creator/3  "Commanded Velocity"
  Subsystem/4(Propeller Efficiency) -> Bus Creator/4  "Commanded Propeller Efficiency"
  Subsystem/5(Fuel Efficiency) -> Bus Creator/5  "Commanded Fuel Mixture"
  Subsystem/6(Flap Angle) -> Bus Creator/6  "Commanded Flap Angle"
  Subsystem/7(Left Brake) -> Bus Creator/7  "Commanded Left Brake"
  Subsystem/8(Right Brake) -> Bus Creator/8  "Commanded Right Brake"
  Subsystem/9(Aileron trim) -> Bus Creator/9  "Commanded Aileron Trim"
  Subsystem/10(Elevator Trim) -> Bus Creator/10  "Commanded Elevator Trim"
  Subsystem/11(Rudder Trim) -> Bus Creator/11  "Commanded Rudder Trim"
  States/1 -> Bus Selector/1, States Out/1
  Waypoint Follower/3 -> Terminator/1
  Waypoint Follower/4 -> Terminator1/1
  Constant/1 -> Waypoint Follower/2
  Constant1/1 -> Waypoint Follower/3
  Mux/1 -> Waypoint Follower/1
  Bus Selector/1 -> Mux/1  "<x>"
  Bus Selector/2 -> Mux/2  "<y>"
  Bus Selector/3 -> Mux/3  "<z>"
  Waypoint Follower/2 -> MATLAB Function/1("heading ")
  Atmosphere/1 -> Atmos/1
  Waypoint Follower/1 -> Subsystem/1(Target)
  MATLAB Function/1(heading) -> Subsystem/2(Desired Heading)
  Radians to Degrees/1 -> Mux/4, Subsystem/3(Heading)
  Bus Selector/4 -> Radians to Degrees/1  "<psi>"

== system DA40_Flight_Model/Correlator Simulation/Subsystem1/Generating GPS and Satellite Measurements1/Truth Model/Navigation1 ==
  Atmosphere : Inport
  Controls : Inport  Port=2
  Constant1 : Constant  Value=DCAM.FVDM.Vehicle.MassProp.Mass
  DA-40 Equations of Motion : Subsystem
  Flight Mechanics and Systems Models : Subsystem
  States : Outport
  wires:
  Flight Mechanics and Systems Models/1(Fb) -> DA-40 Equations of Motion/1(Fb [lb])
  Flight Mechanics and Systems Models/2(Mb) -> DA-40 Equations of Motion/2(Mb [lb-ft])
  Controls/1 -> Flight Mechanics and Systems Models/2(Control Commands)
  Atmosphere/1 -> Flight Mechanics and Systems Models/1(Atmosphere)
  Constant1/1 -> DA-40 Equations of Motion/3(Mass Properties)
  DA-40 Equations of Motion/1(States) -> States/1, Flight Mechanics and Systems Models/3(States)

== system DA40_Flight_Model/Correlator Simulation/Subsystem1/Subsystem2/Subsystem2/Subsystem2 ==
  samplesPerPDI : Inport
  initialCarrierFrequency : Inport  Port=2
  measuredCarrierFrequency : Inport  Port=3
  initialCodeFrequency : Inport  Port=4
  "initialCodePhase " : Inport  Port=5
  measuredCodeFrequency : Inport  Port=6
  chipRate : Inport  Port=7
  dSvClk : Inport  Port=8
  MATLAB Function1 : MATLAB Function  TreatAsAtomicUnit=on
  MATLAB Function4 : MATLAB Function  TreatAsAtomicUnit=on
  samplesPerPDI1 : InportShadow
  sampleVector : Outport
  carrierChangePerSample : Outport  Port=2
  CarrierFrequency : Outport  Port=3
  codeChangePerSample : Outport  Port=4
  initialCodePhase : Outport  Port=5
  wires:
  samplesPerPDI1/1 -> MATLAB Function1/1(samplesPerPDI)
  chipRate/1 -> MATLAB Function1/5(chipRate)
  initialCodeFrequency/1 -> MATLAB Function1/2(initialCodeFrequency)
  measuredCodeFrequency/1 -> MATLAB Function1/4(measuredCodeFrequency)
  MATLAB Function1/1(codeChangePerSample) -> codeChangePerSample/1
  dSvClk/1 -> MATLAB Function1/6(dSvClk)
  "initialCodePhase "/1 -> MATLAB Function1/3("initialCodePhase ")
  MATLAB Function1/2(initialCodePhase) -> initialCodePhase/1
  measuredCarrierFrequency/1 -> MATLAB Function4/3(measuredCarrierFrequency), CarrierFrequency/1
  MATLAB Function4/2(carrierChangePerSample) -> carrierChangePerSample/1
  MATLAB Function4/1(sampleVector) -> sampleVector/1
  initialCarrierFrequency/1 -> MATLAB Function4/2(initialCarrierFrequency)
  samplesPerPDI/1 -> MATLAB Function4/1(samplesPerPDI)

== system DA40_Flight_Model/Correlator Simulation/Subsystem1/Subsystem2/Subsystem3/Subsystem2 ==
  samplesPerPDI : Inport
  initialCarrierFrequency : Inport  Port=2
  measuredCarrierFrequency : Inport  Port=3
  initialCodeFrequency : Inport  Port=4
  "initialCodePhase " : Inport  Port=5
  measuredCodeFrequency : Inport  Port=6
  chipRate : Inport  Port=7
  dSvClk : Inport  Port=8
  MATLAB Function1 : MATLAB Function  TreatAsAtomicUnit=on
  MATLAB Function4 : MATLAB Function  TreatAsAtomicUnit=on
  samplesPerPDI1 : InportShadow
  sampleVector : Outport
  carrierChangePerSample : Outport  Port=2
  CarrierFrequency : Outport  Port=3
  codeChangePerSample : Outport  Port=4
  initialCodePhase : Outport  Port=5
  wires:
  samplesPerPDI/1 -> MATLAB Function4/1(samplesPerPDI)
  initialCarrierFrequency/1 -> MATLAB Function4/2(initialCarrierFrequency)
  MATLAB Function4/1(sampleVector) -> sampleVector/1
  MATLAB Function4/2(carrierChangePerSample) -> carrierChangePerSample/1
  measuredCarrierFrequency/1 -> CarrierFrequency/1, MATLAB Function4/3(measuredCarrierFrequency)
  MATLAB Function1/2(initialCodePhase) -> initialCodePhase/1
  "initialCodePhase "/1 -> MATLAB Function1/3("initialCodePhase ")
  dSvClk/1 -> MATLAB Function1/6(dSvClk)
  MATLAB Function1/1(codeChangePerSample) -> codeChangePerSample/1
  measuredCodeFrequency/1 -> MATLAB Function1/4(measuredCodeFrequency)
  initialCodeFrequency/1 -> MATLAB Function1/2(initialCodeFrequency)
  chipRate/1 -> MATLAB Function1/5(chipRate)
  samplesPerPDI1/1 -> MATLAB Function1/1(samplesPerPDI)

== system DA40_Flight_Model/Extended Kalman Filter/Noise Model/Navigation/Flight Mechanics and Systems Models/Engine + Prop Model ==
  X : Inport
  Control Vector : Inport  Port=2
  Atmosphere : Inport  Port=3
  Bus Selector : BusSelector  OutputSignals=Throttle,Mixture Lever,Prop Lever
  Subsystem : Subsystem
  Engine Thrust : Outport
  Engine Torque : Outport  Port=2
  Prop RPM : Outport  Port=3  PortDimensions=1
  Fuel Flow : Outport  Port=4  PortDimensions=1
  Manifold Pressure : Outport  Port=5  PortDimensions=1
  wires:
  X/1 -> Subsystem/1(X)
  Subsystem/3(Prop RPM) -> Prop RPM/1
  Subsystem/4(Fuel Flow) -> Fuel Flow/1
  Subsystem/5(Manifold Pressure) -> Manifold Pressure/1
  Control Vector/1 -> Bus Selector/1
  Bus Selector/1 -> Subsystem/2(Throttle Setting)  "<Throttle>"
  Bus Selector/2 -> Subsystem/3(Mix)  "<Mixture Lever>"
  Bus Selector/3 -> Subsystem/4(Prop Pitch)  "<Prop Lever>"
  Atmosphere/1 -> Subsystem/5(Atmosphere)
  Subsystem/2(Engine Torque) -> Engine Torque/1
  Subsystem/1(Engine Thrust) -> Engine Thrust/1

== system DA40_Flight_Model/Extended Kalman Filter/Noise Model/Navigation/Flight Mechanics and Systems Models/Gear ==
  State Vector : Inport
  Control Vector : Inport  Port=2
  Friction Coefficients : Inport  Port=3
  " " : MATLAB Function  TreatAsAtomicUnit=on
  Bus Selector : BusSelector  OutputSignals=LeftBrake,RightBrake,Pedal Posn
  Mux : Mux  Inputs=3
  Landing Force : Outport
  Landing Moment : Outport  Port=2
  wires:
  Friction Coefficients/1 -> " "/3(mu)
  State Vector/1 -> " "/2(X)
  " "/1(Ground_Forces) -> Landing Force/1
  " "/2(Ground_Moments) -> Landing Moment/1
  Control Vector/1 -> Bus Selector/1
  Mux/1 -> " "/1(U)
  Bus Selector/1 -> Mux/1  "<LeftBrake>"
  Bus Selector/2 -> Mux/2  "<RightBrake>"
  Bus Selector/3 -> Mux/3  "<Pedal Posn>"

== system DA40_Flight_Model/Extended Kalman Filter/Noise Model/Navigation/Flight Mechanics and Systems Models/Gravity ==
  States : Inport
  Mass Properties : Inport  Port=2
  Constant : Constant  Value=DCAM.FVDM.Vehicle.MassProp.r_cg
  MATLAB Function : MATLAB Function  TreatAsAtomicUnit=on
  Forces due to gravity : Outport
  Moment due to gravity : Outport  Port=2
  wires:
  MATLAB Function/1(F_grav_b) -> Forces due to gravity/1
  States/1 -> MATLAB Function/1(X)
  Mass Properties/1 -> MATLAB Function/2(Mass_Properties)
  MATLAB Function/2(M_grav_b) -> Moment due to gravity/1
  Constant/1 -> MATLAB Function/3(CG)

== system DA40_Flight_Model/Extended Kalman Filter/Noise Model/Navigation/Flight Mechanics and Systems Models/Strip Theory Aero + Propulsive Forces ==
  Atmosphere : Inport
  State Vector : Inport  Port=2
  Control Vector : Inport  Port=3
  Strip Geometry : Inport  Port=4
  Strip_Theory_Modeling : MATLAB Function  TreatAsAtomicUnit=on
  Strip Theory Forces : Outport
  Strip Theory Moments : Outport  Port=2
  wires:
  Atmosphere/1 -> Strip_Theory_Modeling/1(atmos)
  Strip Geometry/1 -> Strip_Theory_Modeling/4(stripGeom)
  Control Vector/1 -> Strip_Theory_Modeling/3(U)
  State Vector/1 -> Strip_Theory_Modeling/2(X)
  Strip_Theory_Modeling/1(Strip_Theory_Forces) -> Strip Theory Forces/1
  Strip_Theory_Modeling/2(Strip_Theory_Moments) -> Strip Theory Moments/1

== system DA40_Flight_Model/Extended Kalman Filter/Noise Model/Navigation/Flight Mechanics and Systems Models/Sum of Forces + Noise ==
  Engine : Inport
  Aero : Inport  Port=2
  Landing : Inport  Port=3
  Gravity : Inport  Port=4
  Add : Sum  Inputs=++++
  Add1 : Sum
  Add3 : Sum
  Add4 : Sum
  Band-Limited White Noise : simulink/Sources/Band-Limited White Noise  Cov=DCAM.FVDM.gravity.force  Ts=DCAM.FVDM.gravity.forceTS  seed=DCAM.currentSeed
  Band-Limited White Noise2 : simulink/Sources/Band-Limited White Noise  Cov=DCAM.FVDM.aero.force  Ts=DCAM.FVDM.aero.forceTS  seed=DCAM.currentSeed
  Band-Limited White Noise3 : simulink/Sources/Band-Limited White Noise  Cov=DCAM.FVDM.engine.force  Ts=DCAM.FVDM.engine.forceTS  seed=DCAM.currentSeed
  F_b : Outport
  wires:
  Add/1 -> F_b/1
  Gravity/1 -> Add1/1
  Add1/1 -> Add/4
  Band-Limited White Noise/1 -> Add1/2
  Landing/1 -> Add/3
  Band-Limited White Noise2/1 -> Add3/2
  Add3/1 -> Add/2
  Aero/1 -> Add3/1
  Band-Limited White Noise3/1 -> Add4/2
  Add4/1 -> Add/1
  Engine/1 -> Add4/1

== system DA40_Flight_Model/Extended Kalman Filter/Noise Model/Navigation/Flight Mechanics and Systems Models/Sum of Moments + Noise ==
  Engine : Inport
  Aero : Inport  Port=2
  Landing : Inport  Port=3
  Gravity : Inport  Port=4
  Add : Sum  Inputs=++++
  Add1 : Sum
  Add3 : Sum
  Add4 : Sum
  Band-Limited White Noise : simulink/Sources/Band-Limited White Noise  Cov=DCAM.FVDM.gravity.moment  Ts=DCAM.FVDM.gravity.momentTS  seed=DCAM.currentSeed
  Band-Limited White Noise2 : simulink/Sources/Band-Limited White Noise  Cov=DCAM.FVDM.aero.moment  Ts=DCAM.FVDM.aero.momentTS  seed=DCAM.currentSeed
  Band-Limited White Noise3 : simulink/Sources/Band-Limited White Noise  Cov=DCAM.FVDM.engine.moment  Ts=DCAM.FVDM.engine.momentTS  seed=DCAM.currentSeed
  M_b : Outport
  wires:
  Engine/1 -> Add4/1
  Add4/1 -> Add/1
  Band-Limited White Noise3/1 -> Add4/2
  Aero/1 -> Add3/1
  Add3/1 -> Add/2
  Band-Limited White Noise2/1 -> Add3/2
  Landing/1 -> Add/3
  Band-Limited White Noise/1 -> Add1/2
  Add1/1 -> Add/4
  Gravity/1 -> Add1/1
  Add/1 -> M_b/1

== system DA40_Flight_Model/Correlator Simulation/Subsystem1/Generating GPS and Satellite Measurements/Truth Model/Control/Send To Workspace ==
  States : Inport
  Constant : Constant  Value=0
  Demux : Demux  Outputs=2
  Flat Earth to LLA : aerolibtransform2/Flat Earth to LLA  units=Metric (MKS)  ptype=Earth (WGS84)  F=1/298.257223563  R=6378137  refPosPort=off  LL0=DCAM.FVDM.refLL  psi=0
  Mux : Mux  Inputs=3
  Selector1 : Selector  InputPortWidth=12  IndexOptions=Index vector (dialog)  Indices=[7:9]  OutputSizes=1
  To Workspace1 : ToWorkspace  VariableName=trueLONG  SampleTime=-1
  To Workspace2 : ToWorkspace  VariableName=trueALT  SampleTime=-1
  To Workspace6 : ToWorkspace  VariableName=trueLAT  SampleTime=-1
  LLA : Outport
  States Out : Outport  Port=2
  wires:
  States/1 -> States Out/1, Selector1/1
  Selector1/1 -> Flat Earth to LLA/1
  Constant/1 -> Flat Earth to LLA/2
  Flat Earth to LLA/2 -> Mux/3, To Workspace2/1
  Flat Earth to LLA/1 -> Demux/1
  Demux/1 -> Mux/1, To Workspace6/1
  Demux/2 -> Mux/2, To Workspace1/1
  Mux/1 -> LLA/1
